simulink model "BouncingBall"  (R2021a)
settings: Solver=VariableStepAuto  StartTime=0.0  StopTime=10.0  RelTol=1e-3
settings Model: Creator=jiaweichen  LastModifiedBy=jiaweichen

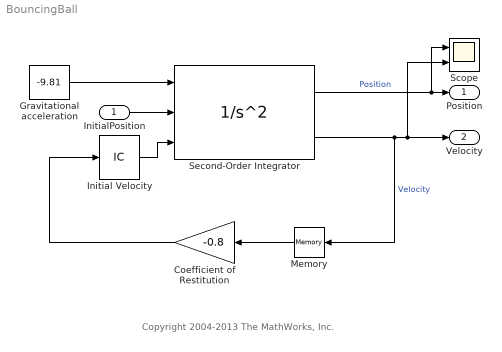
== system BouncingBall ==
  note: Copyright 2004-2013 The MathWorks, Inc.
  InitialPosition : Inport
  Coefficient of Restitution : Gain  Gain=-0.8
  Gravitational acceleration : Constant  Value=-9.81  OutDataTypeStr=double
  "Initial Velocity " : InitialCondition  Value=15
  Memory : Memory
  Scope : Scope  NumInputPorts=2
  Second-Order Integrator : SecondOrderIntegrator  ICSourceX=external  ICX=10.0  LimitX=on  LowerLimitX=0.0  StateNameX='Position'  ICSourceDXDT=external  StateNameDXDT='Velocity'  ReinitDXDTwhenXreachesSaturation=on
  Position : Outport
  Velocity : Outport  Port=2
  wires:
  Gravitational acceleration/1 -> Second-Order Integrator/1
  Second-Order Integrator/1 -> Scope/1, Position/1  "Position"
  "Initial Velocity "/1 -> Second-Order Integrator/3
  Second-Order Integrator/2 -> Velocity/1, Scope/2, Memory/1  "Velocity"
  Memory/1 -> Coefficient of Restitution/1
  Coefficient of Restitution/1 -> "Initial Velocity "/1
  InitialPosition/1 -> Second-Order Integrator/2
